simulink model "reg_z_calk"  (R2021a)
settings: Solver=VariableStepAuto  StartTime=0.0  StopTime=1000  RelTol=1e-3
values from neighbouring files (symbols this model uses):
  k1 = k(1,1)    [liczenie_k.m]    (also in skrypt_k_i_l.m; zad4.m; zad_dod.m = K(1))
  k2 = k(1,2)    [liczenie_k.m]    (also in skrypt_k_i_l.m; zad4.m; zad_dod.m = K(2))
  k3 = k(1,3)    [liczenie_k.m]    (also in skrypt_k_i_l.m; zad4.m; zad_dod.m = K(3))
  ke = K(4)    [zad_dod.m]
  mult = 1.3    [zad_dod.m]
settings Model: Creator=ADMIN  LastModifiedBy=ADMIN

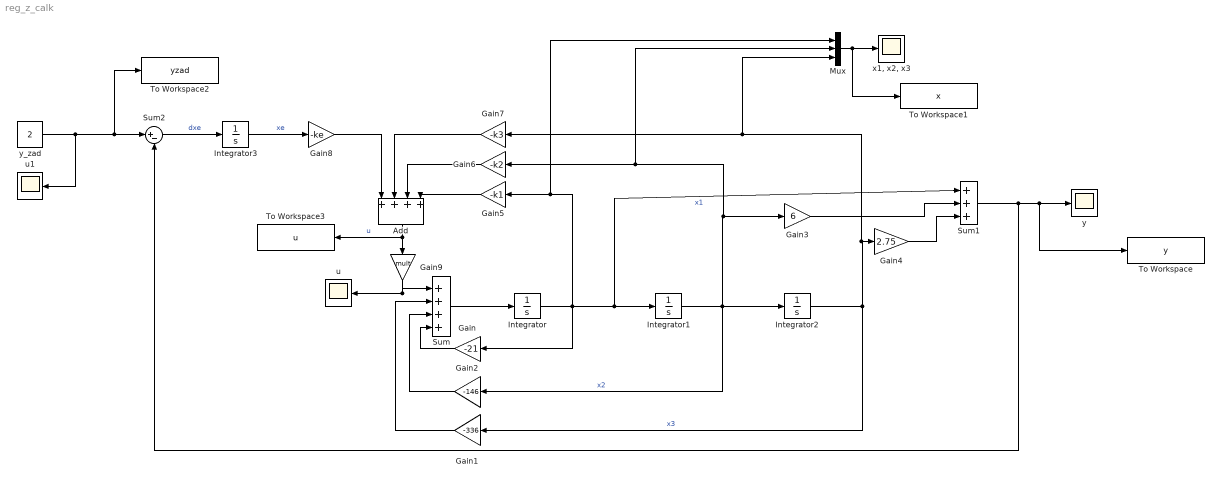
== system reg_z_calk ==
  Add : Sum  Inputs=++++
  Gain : Gain  Gain=-21
  Gain1 : Gain  Gain=-336
  Gain2 : Gain  Gain=-146
  Gain3 : Gain  Gain=6
  Gain4 : Gain  Gain=2.75
  Gain5 : Gain  Gain=-k1
  Gain6 : Gain  Gain=-k2
  Gain7 : Gain  Gain=-k3
  Gain8 : Gain  Gain=-ke
  Gain9 : Gain  Gain=mult
  Integrator : Integrator  InitialCondition=1
  Integrator1 : Integrator  InitialCondition=2
  Integrator2 : Integrator  InitialCondition=4
  Integrator3 : Integrator
  Mux : Mux  Inputs=3
  Sum : Sum  Inputs=|++++
  Sum1 : Sum  Inputs=|+++
  Sum2 : Sum  Inputs=|+-
  To Workspace : ToWorkspace  VariableName=y  SaveFormat=Structure With Time  SampleTime=-1
  To Workspace1 : ToWorkspace  VariableName=x  SaveFormat=Structure With Time  SampleTime=-1
  To Workspace2 : ToWorkspace  VariableName=yzad  SaveFormat=Structure With Time  SampleTime=-1
  To Workspace3 : ToWorkspace  VariableName=u  SaveFormat=Structure With Time  SampleTime=-1
  u : Scope
  u1 : Scope
  "x1, x2, x3" : Scope
  y : Scope
  y_zad : Constant  Value=2  SampleTime=-1
  wires:
  Integrator/1 -> Mux/1, Gain5/1, Sum1/1, Integrator1/1, Gain/1  "x1"
  Gain3/1 -> Sum1/2
  Integrator2/1 -> Gain1/1, Mux/3, Gain7/1, Gain4/1  "x3"
  Integrator1/1 -> Mux/2, Gain6/1, Gain3/1, Gain2/1, Integrator2/1  "x2"
  Sum/1 -> Integrator/1
  Gain4/1 -> Sum1/3
  Mux/1 -> To Workspace1/1, "x1, x2, x3"/1
  Sum1/1 -> Sum2/2, To Workspace/1, y/1
  Gain1/1 -> Sum/2
  Gain2/1 -> Sum/3
  Gain/1 -> Sum/4
  y_zad/1 -> u1/1, To Workspace2/1, Sum2/1
  Sum2/1 -> Integrator3/1  "dxe"
  Integrator3/1 -> Gain8/1  "xe"
  Gain5/1 -> Add/4
  Gain6/1 -> Add/3
  Gain7/1 -> Add/2
  Gain8/1 -> Add/1
  Add/1 -> To Workspace3/1, Gain9/1  "u"
  Gain9/1 -> u/1, Sum/1
